simulink model "areverse_park_clark"  (R2015a)
settings: Solver=ode45  StartTime=0.0  StopTime=40/1000  RelTol=1e-3
settings Model: Creator=Windows 10  LastModifiedBy=Windows 10

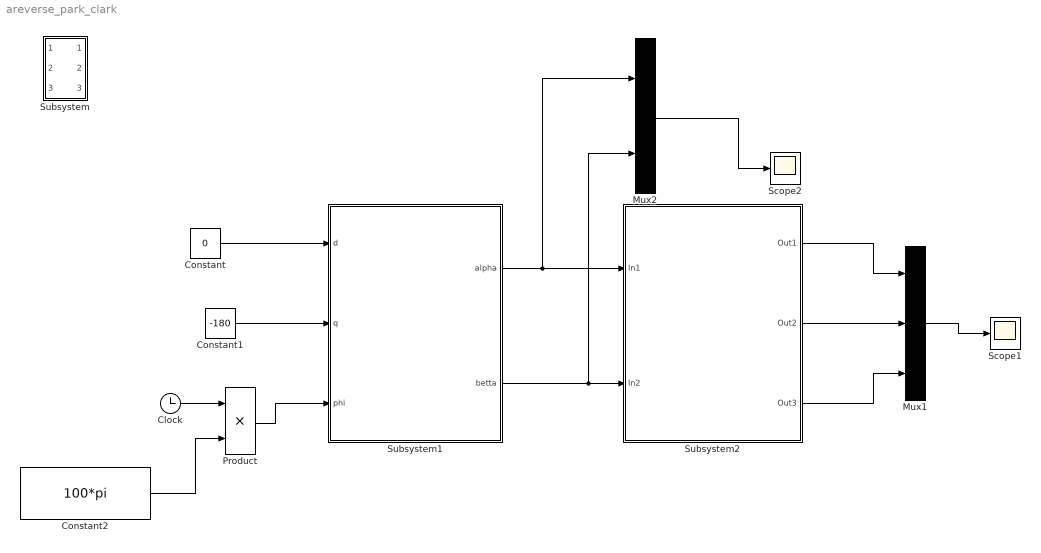
== system areverse_park_clark ==
  Clock : Clock
  Constant : Constant  Value=0
  Constant1 : Constant  Value=-180
  Constant2 : Constant  Value=100*pi
  Mux1 : Mux  Inputs=3
  Mux2 : Mux  Inputs=2
  Product : Product
  Scope1 : Scope
  Scope2 : Scope
  Subsystem : Subsystem
  Subsystem1 : Subsystem
  Subsystem2 : Subsystem
  wires:
  Clock/1 -> Product/1
  Constant2/1 -> Product/2
  Mux1/1 -> Scope1/1
  Subsystem1/1(alpha) -> Mux2/1, Subsystem2/1(In1)
  Product/1 -> Subsystem1/3(phi)
  Constant/1 -> Subsystem1/1(d)
  Constant1/1 -> Subsystem1/2(q)
  Subsystem1/2(betta) -> Mux2/2, Subsystem2/2(In2)
  Subsystem2/2(Out2) -> Mux1/2
  Subsystem2/1(Out1) -> Mux1/1
  Subsystem2/3(Out3) -> Mux1/3
  Mux2/1 -> Scope2/1

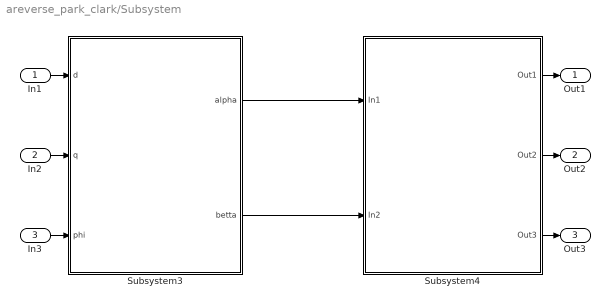
== system areverse_park_clark/Subsystem ==
  In1 : Inport
  In2 : Inport  Port=2
  In3 : Inport  Port=3
  Subsystem3 : Subsystem
  Subsystem4 : Subsystem
  Out1 : Outport
  Out2 : Outport  Port=2
  Out3 : Outport  Port=3
  wires:
  Subsystem3/1(alpha) -> Subsystem4/1(In1)
  Subsystem3/2(betta) -> Subsystem4/2(In2)
  In2/1 -> Subsystem3/2(q)
  In1/1 -> Subsystem3/1(d)
  In3/1 -> Subsystem3/3(phi)
  Subsystem4/1(Out1) -> Out1/1
  Subsystem4/2(Out2) -> Out2/1
  Subsystem4/3(Out3) -> Out3/1

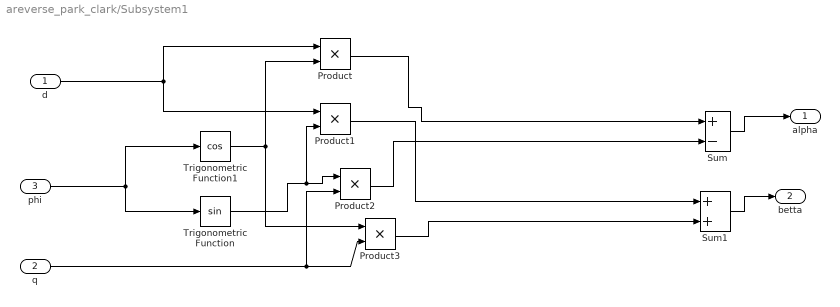
== system areverse_park_clark/Subsystem1 ==
  d : Inport
  q : Inport  Port=2
  phi : Inport  Port=3
  Product{,1..3} (4 alike) : Product
  Sum : Sum  Inputs=+-
  Sum1 : Sum
  Trigonometric Function : Trigonometry
  Trigonometric Function1 : Trigonometry  Operator=cos
  alpha : Outport
  betta : Outport  Port=2
  wires:
  Sum/1 -> alpha/1
  Sum1/1 -> betta/1
  phi/1 -> Trigonometric Function/1, Trigonometric Function1/1
  Product/1 -> Sum/1
  Product1/1 -> Sum1/1
  Product2/1 -> Sum/2
  Product3/1 -> Sum1/2
  q/1 -> Product2/2, Product3/2
  Trigonometric Function/1 -> Product1/2, Product2/1
  Trigonometric Function1/1 -> Product3/1, Product/2
  d/1 -> Product1/1, Product/1

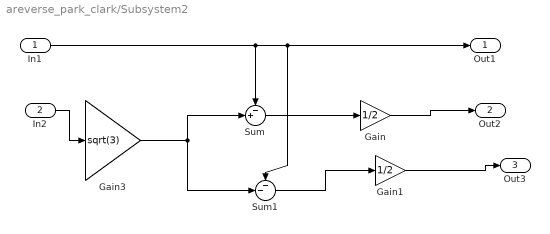
== system areverse_park_clark/Subsystem2 ==
  In1 : Inport
  In2 : Inport  Port=2
  Gain : Gain  Gain=1/2
  Gain1 : Gain  Gain=1/2
  Gain3 : Gain  Gain=sqrt(3)
  Sum : Sum  Inputs=-+|
  Sum1 : Sum  Inputs=--|
  Out1 : Outport
  Out2 : Outport  Port=2
  Out3 : Outport  Port=3
  wires:
  Gain/1 -> Out2/1
  Gain1/1 -> Out3/1
  In2/1 -> Gain3/1
  Gain3/1 -> Sum/2, Sum1/2
  In1/1 -> Sum1/1, Out1/1, Sum/1
  Sum/1 -> Gain/1
  Sum1/1 -> Gain1/1

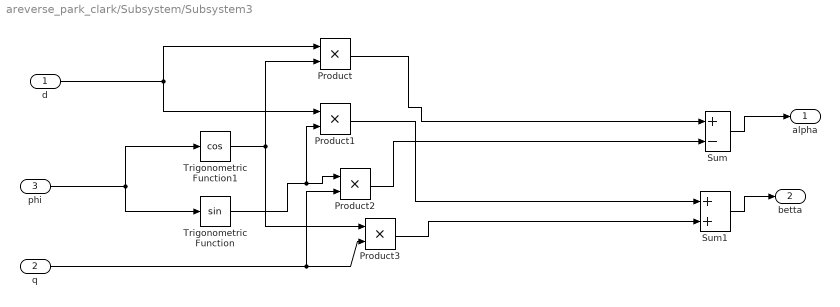
== system areverse_park_clark/Subsystem/Subsystem3 ==
  d : Inport
  q : Inport  Port=2
  phi : Inport  Port=3
  Product{,1..3} (4 alike) : Product
  Sum : Sum  Inputs=+-
  Sum1 : Sum
  Trigonometric Function : Trigonometry
  Trigonometric Function1 : Trigonometry  Operator=cos
  alpha : Outport
  betta : Outport  Port=2
  wires:
  d/1 -> Product/1, Product1/1
  Trigonometric Function1/1 -> Product/2, Product3/1
  Trigonometric Function/1 -> Product2/1, Product1/2
  q/1 -> Product3/2, Product2/2
  Product3/1 -> Sum1/2
  Product2/1 -> Sum/2
  Product1/1 -> Sum1/1
  Product/1 -> Sum/1
  phi/1 -> Trigonometric Function1/1, Trigonometric Function/1
  Sum1/1 -> betta/1
  Sum/1 -> alpha/1

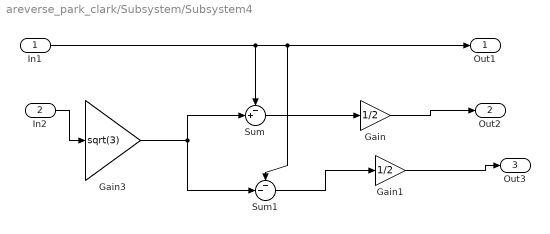
== system areverse_park_clark/Subsystem/Subsystem4 ==
  In1 : Inport
  In2 : Inport  Port=2
  Gain : Gain  Gain=1/2
  Gain1 : Gain  Gain=1/2
  Gain3 : Gain  Gain=sqrt(3)
  Sum : Sum  Inputs=-+|
  Sum1 : Sum  Inputs=--|
  Out1 : Outport
  Out2 : Outport  Port=2
  Out3 : Outport  Port=3
  wires:
  Sum1/1 -> Gain1/1
  Sum/1 -> Gain/1
  In1/1 -> Sum/1, Out1/1, Sum1/1
  Gain3/1 -> Sum1/2, Sum/2
  In2/1 -> Gain3/1
  Gain1/1 -> Out3/1
  Gain/1 -> Out2/1
